simulink model "model2"  (R2024b)
settings: Solver=ode45  StartTime=0.0  StopTime=100  RelTol=1e-3  AbsTol=1e-6
values from neighbouring files (symbols this model uses):
  A = media*ones(2001, 1)    [Codice.m]    (also in creAB.m = mdiagonal(A,[0 1;a1(i) a2(i)]))
  B = mdiagonal(B,[0;b1(i)])    [creAB.m]
settings Model: Creator=tschauer  LastModifiedBy=User
settings DataIOCC: SaveFormat=Array  SignalLoggingSaveFormat=ModelDataLogs  SaveOutput=off  SignalLogging=off  DSMLogging=off  SaveTime=off  ReturnWorkspaceOutputs=off
settings OptimizationCC: BlockReduction=off  BooleanDataType=off
settings DebuggingCC: SaveWithParameterizedLinksMsg=none  UnderspecifiedInitializationDetection=Classic  MergeDetectMultiDrivingBlocksExec=none  SignalResolutionControl=TryResolveAllWithWarning  MultiTaskDSMMsg=warning  MultiTaskCondExecSysMsg=none  UnconnectedInputMsg=warning  UnconnectedOutputMsg=warning  UnconnectedLineMsg=warning
settings HardwareCC: TargetUnknown=on
settings ModelReferenceCC: PropagateSignalLabelsOutOfModel=off
settings GRTTargetCC: CombineOutputUpdateFcns=off  GRTInterface=on

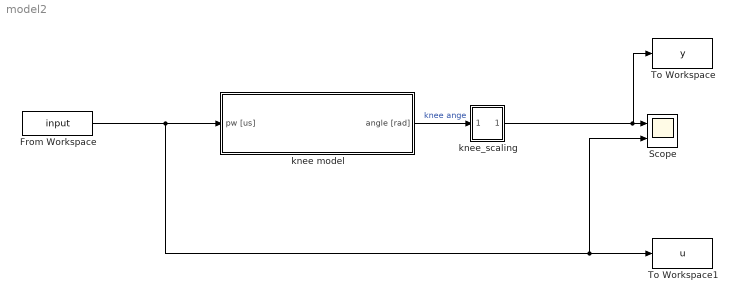
== system model2 ==
  From Workspace : FromWorkspace  VariableName=input  SampleTime=0.05  Interpolate=off  ZeroCross=off  OutputAfterFinalValue=Setting to zero
  Scope : Scope  NumInputPorts=2
  To Workspace : ToWorkspace  VariableName=y  SampleTime=0.05
  To Workspace1 : ToWorkspace  VariableName=u  SampleTime=0.05
  knee model : Subsystem  mask{freq=20, qk0=1.54248, act0=[0 0 0 0 0 0    0 0 0.0 0 0.0 0   0 0 0 0 0 0 ]}
      mask prompts: freq "frequency:"; qk0 "initial knee angle:"; act0 "initial states for musle activation:"
      mask init:
      | [A,B]=creAB;
      mask Display: disp('Knee model')
  knee_scaling : Subsystem
  wires:
  knee model/1(angle [rad]) -> knee_scaling/1(in_1)  "knee ange"
  knee_scaling/1(knee_angle_[deg]) -> To Workspace/1, Scope/1
  From Workspace/1 -> Scope/2, To Workspace1/1, knee model/1(pw [us])

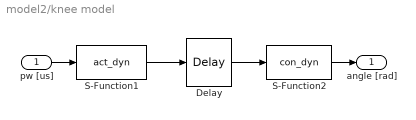
== system model2/knee model ==
  pw [us] : Inport
  Delay : TransportDelay  DelayTime=0.025  InitialOutput=act0(1:2:17)
  S-Function1 : S-Function  FunctionName=act_dyn  Parameters=act0,freq,A,B  SFunctionDeploymentMode=off  EnableBusSupport=off
  S-Function2 : S-Function  FunctionName=con_dyn  Parameters=qk0  SFunctionDeploymentMode=off  EnableBusSupport=off
  angle [rad] : Outport  InitialOutput=0
  wires:
  S-Function1/1 -> Delay/1
  pw [us]/1 -> S-Function1/1
  S-Function2/1 -> angle [rad]/1
  Delay/1 -> S-Function2/1

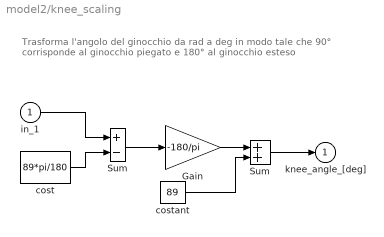
== system model2/knee_scaling ==
  note: Trasforma l'angolo del ginocchio da rad a deg in modo tale che
      | 90° corrisponde al ginocchio piegato e 180° al ginocchio esteso
  in_1 : Inport
  Gain : Gain  Gain=-180/pi  SaturateOnIntegerOverflow=on  OutDataTypeStr=Inherit: Same as input  ParamDataTypeStr=Inherit: Same as input
  "Sum " : Sum  Inputs=+-  InputSameDT=on  SaturateOnIntegerOverflow=on  OutDataTypeStr=Inherit: Same as first input
  "Sum " : Sum  InputSameDT=on  SaturateOnIntegerOverflow=on  OutDataTypeStr=Inherit: Same as first input
  cost : Constant  Value=89*pi/180
  "costant " : Constant  Value=89
  knee_angle_[deg] : Outport  InitialOutput=0
  wires:
  "Sum "/1 -> knee_angle_[deg]/1
  in_1/1 -> "Sum "/1
  cost/1 -> "Sum "/2
  "Sum "/1 -> Gain/1
  Gain/1 -> "Sum "/1
  "costant "/1 -> "Sum "/2
